simulink model "main"  (R2020b)
settings: Solver=ode23tb  StartTime=0.0  StopTime=20  FixedStep=0.0005  MaxStep=0.005  RelTol=1e-3  AbsTol=1e-3
StartFcn:
  | tic;
StopFcn:
  | Elapsed_Sim_Time = toc;
  | disp(['Elapsed Sim Time = ' num2str(Elapsed_Sim_Time)]);
model workspace (MATLAB code in the model file):
  | floor_l = 1.0900;
  | floor_d = 0.0100;
  | 
  | % PART
  | model_idx = 0;
  | model_dims = [0.06 0.06 0.06;
  |      0.02 0.05 0.07;
  |      0.04 0.04 0.10;
  |      0.05 0.05 0.05;
  |      0.10 0.08 0.08];
  | % distance between models on the conveyor belt
  | model_d = 0.12;
  | % distance to push models forwards in the -y dir (towards the box)
  | model_push = 0.2;
  | 
  | % BELT
  | belt_w = 0.1000;
  | belt_l = 1.2000;
  | belt_h = 0.0200;
  | belt_in_offset = [0 0.8000 0.0100];
  | 
  | container_belt_h = 0.02;
  | container_belt_l = 2.0;
  | container_belt_w = 0.2;
  | container_belt_offset = [-0.5050 0 -0.020];
  | 
  | belt_spd = 0.1;
  | 
  | % Model
  | cube_d = 0.06;
  | cube_z_off = belt_in_offset(3) + (container_belt_h / 2) + 0.001;
  | cube_z_offs = (model_dims(:,3) / 2) + cube_z_off;
  | 
  | % Container dimensions
  | % len, width, height are INTERNAL (Changed because most things were using internal anyway and it's 4am and we just need a working demo)
  | % Dimensions
  | container_len = 0.2;
  | container_width = 0.15;
  | container_height = 0.15;
  | container_thickness = 0.005;
  | 
  | 
  | % ????
  | cube_con_rsph = 0.003;
  | 
  | cube_con_k = 1000000;
  | cube_con_b = 1000;
  | 
  | finger_con_x = 0.01;
  | finger_con_y = 0.01;
  | finger_con_z = 5e-4;
  | finger_con_rsph = 5.0000e-04;
  | finger_con_muk = 0.05;
  | finger_con_mus = 0.07;
  | finger_con_vth = 1e-3;
  | 
  | finger_l = 0.4;
  | finger_w = 0.03;
  | finger_t = 0.01;
undefined symbols (not defined in the file): Bottom, Extr_Data_LinkHoles, Part1, Part2, Part3, Part4, Part5, point1, point2, point3, Side1, Side2, Side3, Side4, X, Y, Z
libraries: sm_lib x113, nesl_utility x35, Parts_Lib x10, Contact_Forces_Lib x6, sm_delta_robot_lib x1
(part 3 of 5)

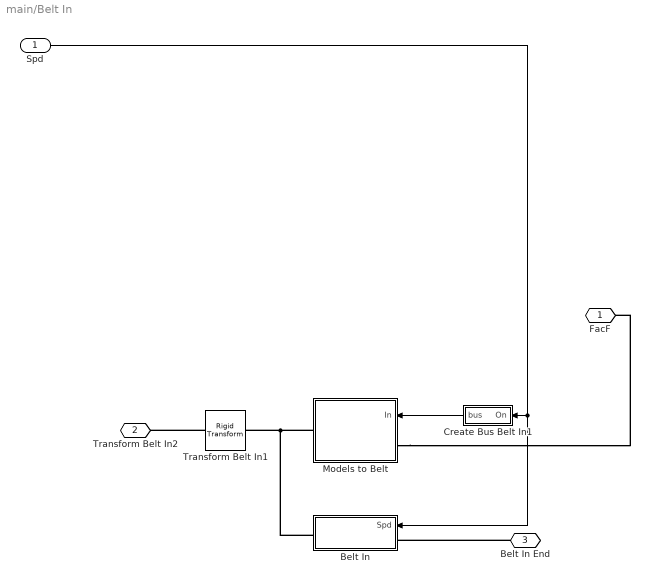
== system main/Belt In ==
  Spd : Inport
  Belt In : Subsystem  Tag=CustomStyle  mask(Conveyor Belt, 5 Rollers){belt_l=belt_l, belt_d=belt_h, belt_w=belt_w, roller_clr=[1 1 1], ctrrefnorm_popup=+Z}
      mask prompts: belt_l "Conveyor Length (m)"; belt_d "Conveyor Depth (m)"; belt_w "Conveyor Width (m)"; roller_clr "Roller Color (rgb)"; ctrrefnorm_popup "Center Reference Frame, Normal Axis"
      mask help: Models a conveyor belt. Input signal is belt speed which only affects roller rotational speed in animation.
      mask init:
      | temp_curblk = gcb;
      | if strcmp(get_param(temp_curblk,'ctrrefnorm_popup'),'+Z')
      |     set_param([temp_curblk '/Transform Contact Ref'],'RotationSequenceAngles','[-90 0 0]');
      | elseif strcmp(get_param(temp_curblk,'ctrrefnorm_popup'),'+X')
      |     set_param([temp_curblk '/Transform Contact Ref'],'RotationSequenceAngles','[0 0 90]');
      | end
      | clear temp_curblk
      mask TypeOptions ctrrefnorm_popup: +Z | +X
  Create Bus Belt In1 : Subsystem
  Models to Belt : Subsystem
  Transform Belt In1 : sm_lib/Frames and Transforms/Rigid Transform  TranslationMethod=Cartesian  TranslationStandardOffset=0  TranslationLengthUnit=m  TranslationStandardAxis=+Y  TranslationCartesianOffset=belt_in_offset  TranslationROffset=0  TranslationROffsetUnits=m  TranslationZOffset=0  TranslationZOffsetUnits=m  TranslationThetaOffset=0  TranslationThetaOffsetUnits=deg  RotationMethod=StandardAxis  RotationAngleUnits=deg  RotationStandardAxis=+Z  RotationAngle=-90  RotationArbitraryAxis=[0 0 1]  FollAlignAxisA=+X  BaseAlignAxisA=+Y  FollAlignAxisB=+Y  BaseAlignAxisB=+Z  RotationSequenceAxes=FollowerAxes  RotationSequence=XYX  RotationSequenceAngles=[0 0 0]  RotationSequenceAnglesUnits=deg  RotationMatrix=[1 0 0; 0 1 0; 0 0 1]
  FacF : PMIOPort  Side=Right
  Transform Belt In2 : PMIOPort  Port=2  Side=Left
  Belt In End : PMIOPort  Port=3  Side=Right
  wires:
  Create Bus Belt In1/1(bus) -> Models to Belt/1(In)
  Spd/1 -> Belt In/1(Spd), Create Bus Belt In1/1(On)
  connections:
  Transform Belt In1/LConn1 -- Transform Belt In2/RConn1
  Models to Belt/RConn1 -- Belt In/RConn1 -- Transform Belt In1/RConn1
  Models to Belt/LConn1 -- FacF/RConn1
  Belt In End/RConn1 -- Belt In/LConn1

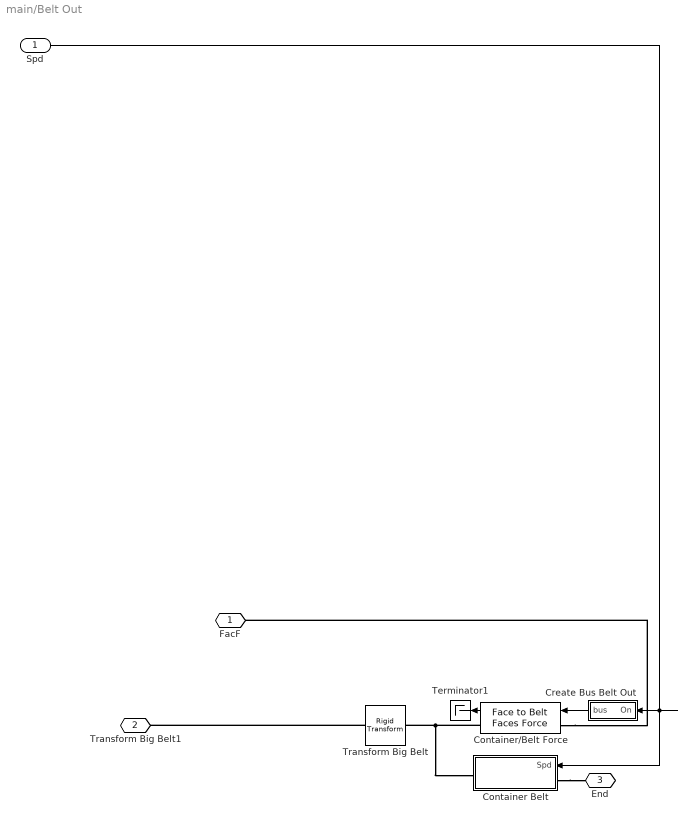
== system main/Belt Out ==
  Spd : Inport
  Container Belt : Subsystem  Tag=CustomStyle  mask(Conveyor Belt, 5 Rollers){belt_l=container_belt_l, belt_d=container_belt_h, belt_w=container_belt_w, roller_clr=[1 1 1], ctrrefnorm_popup=+Z}
      mask prompts: belt_l "Conveyor Length (m)"; belt_d "Conveyor Depth (m)"; belt_w "Conveyor Width (m)"; roller_clr "Roller Color (rgb)"; ctrrefnorm_popup "Center Reference Frame, Normal Axis"
      mask help: Models a conveyor belt. Input signal is belt speed which only affects roller rotational speed in animation.
      mask init: same as main/Belt In/Belt In
      mask TypeOptions ctrrefnorm_popup: +Z | +X
  Container/Belt Force : Contact_Forces_Lib/3D/Composite Forces/Face to Belt Faces Force  PlaB_x=container_belt_l  PlaB_y=container_belt_w  PlaB_z=container_belt_h/2  FacF_x=container_len  FacF_y=container_width  FacF_z=container_thickness/2  FacF_rSph=cube_con_rsph  force_law_pla2pla=Linear  k_contact_pla2pla=stff  b_contact_pla2pla=dmp  pen_full_damp_F_pla2pla=1e-4  pen_exponent_pla2pla=1  friction_law_pla2pla=Stick-Slip Continuous  mu_kinetic_pla2pla=0.5  mu_static_pla2pla=0.7  v_thr_pla2pla=0.001  vis_on_pla2pla=off  vis_opc_en_box2box=0  vis_len_plaLz=0.0005  vis_clr=[0.9 0.2 0.2]  vis_opc=0.7
      link override Sphere to Plane Force Enabled nz1/Forces/Ff/Friction Law/Stick-Slip C /Coefficient of Friction vs Velocity: BeginIndexSearchUsingPreviousIndexResult=on
      link override Sphere to Plane Force Enabled nz2/Forces/Ff/Friction Law/Stick-Slip C /Coefficient of Friction vs Velocity: BeginIndexSearchUsingPreviousIndexResult=on
      link override Sphere to Plane Force Enabled nz3/Forces/Ff/Friction Law/Stick-Slip C /Coefficient of Friction vs Velocity: BeginIndexSearchUsingPreviousIndexResult=on
      settings: SourceProductName=Simscape Multibody Contact Forces Library
  Create Bus Belt Out : Subsystem
  Terminator1 : Terminator
  Transform Big Belt : sm_lib/Frames and Transforms/Rigid Transform  TranslationMethod=Cartesian  TranslationStandardOffset=0  TranslationLengthUnit=m  TranslationStandardAxis=+Y  TranslationCartesianOffset=container_belt_offset  TranslationROffset=0  TranslationROffsetUnits=m  TranslationZOffset=0  TranslationZOffsetUnits=m  TranslationThetaOffset=0  TranslationThetaOffsetUnits=deg  RotationMethod=StandardAxis  RotationAngleUnits=deg  RotationStandardAxis=+Z  RotationAngle=180  RotationArbitraryAxis=[0 0 1]  FollAlignAxisA=+X  BaseAlignAxisA=+Y  FollAlignAxisB=+Y  BaseAlignAxisB=+Z  RotationSequenceAxes=FollowerAxes  RotationSequence=XYX  RotationSequenceAngles=[0 0 0]  RotationSequenceAnglesUnits=deg  RotationMatrix=[1 0 0; 0 1 0; 0 0 1]
  FacF : PMIOPort  Side=Right
  Transform Big Belt1 : PMIOPort  Port=2  Side=Left
  End : PMIOPort  Port=3  Side=Left
  wires:
  Spd/1 -> Container Belt/1(Spd), Create Bus Belt Out/1(On)
  Create Bus Belt Out/1(bus) -> Container/Belt Force/1
  Container/Belt Force/1 -> Terminator1/1
  connections:
  Transform Big Belt/LConn1 -- Transform Big Belt1/RConn1
  Container/Belt Force/RConn1 -- Container Belt/RConn1 -- Transform Big Belt/RConn1
  Container Belt/LConn1 -- End/RConn1
  Container/Belt Force/LConn1 -- FacF/RConn1

== system main/Config ==
  Floor : sm_lib/Body Elements/Brick Solid  Commented=on  GraphicAmbientColor=[0.15 0.15 0.15 1.0]  BasedOnType=Density  BrickDimensions=[floor_l floor_l floor_d]  BrickDimensionUnits=m  CenterOfMass=[0 0 0]  CenterOfMassUnits=m  GraphicDiffuseColor=[0.8 0.8 0.8]  Density=100  DensityUnits=kg/m^3  DoExposeReferenceFrame=on  GraphicEmissiveColor=[0.0 0.0 0.0 1.0]  ExportEntireGeometry=off  SerializedFrames=<Frames><Frame><Id>Frame1</Id><Value><Name>T</Name><Origin><Source>GeometricFeature</Source><FeatureName>+z surface</FeatureName></Origin><PrimaryAxis><DefinedDirection>+Z</DefinedDirection><Source>ReferenceFrame</Source><SourceDirection>+Z</SourceDirection><FeatureName></FeatureName></PrimaryAxis><SecondaryAxis><DefinedDirection>+X</DefinedDirection><Source>ReferenceFrame</Source><SourceDirection>+X</SourceDirection><FeatureName></FeatureName></SecondaryAxis></Value></Frame></Frames>  MarkerShape=Sphere  MarkerSize=10  GraphicType=FromGeometry  InertiaType=CalculateFromGeometry  Mass=1  MassUnits=kg  MomentsOfInertia=[1 1 1]  MomentsOfInertiaUnits=kg*m^2  GraphicOpacity=1.0  ProductsOfInertia=[1 1 1]  ProductsOfInertiaUnits=kg*m^2  GraphicShininess=75  GraphicSpecularColor=[0.5 0.5 0.5 1.0]  GraphicVisPropType=SimpleVisualProperties
  Mechanism Configuration : sm_lib/Utilities/Mechanism Configuration  UniformGravity=Constant  GravityVector=[0 0 -9.80665]  GravityVectorUnits=m/s^2  GravityUnits=m/s^2  LinearizationDelta=0.001  JointModeTransitionNonlinearIterations=2
  Solver Configuration : nesl_utility/Solver Configuration  PhysicalDomain=network_engine_domain  SubClassName=solver  LeftPortType=input  RightPortType=generic  Tones=[]  Harmonics=[]  SimulateNoise=off  Profile=off  UseLocalSampling=off  EnableSwitchedLinearOptims=on  FrequencyDomain=off  UseCCode=off  RelTol=0.001  AbsTol=1e-06  MinStep=1e-09  ToWorkspace=off  RevertToSquareIcSolve=off  NumHomotopyIterations=100  PhasorMode=off  PhasorModeNumHarmonics=1  DoDC=off  ResidualTolerance=1e-05  UseLocalSolver=off  LocalSolverChoice=NE_BACKWARD_EULER_ADVANCER  LocalSolverSampleTime=0.0001  DoFixedCost=off  MaxNonlinIter=3  MaxModeIter=2  ComputeImpulses=on  ImpulseIterations=2  LinearAlgebra=auto  EquationFormulation=NE_TIME_EF  DelaysMemoryBudget=1024  AutomaticFiltering=on  FilteringTimeConstant=0.001  PartitionStorageMethod=AS_NEEDED  PartitionMemoryBudget=1024  PartitionMethod=FAST
  C : PMIOPort  Side=Right
  connections:
  C/RConn1 -- Floor/RConn1 -- Solver Configuration/RConn1 -- Mechanism Configuration/RConn1

== system main/Contacts Models Container ==
  Contacts Model-Container1 : Subsystem  mask{k=500, b=10, mus=0.4, muk=0.4}
      mask prompts: k "Stiffness (N/m)"; b "Dampink (N/(m/s))"; mus "Coefficient of Static Friction"; muk "Coefficient of Dynamic Friction"
      mask DialogControl Control2 Prompt: Force Parameters
  Contacts Model-Container2 : Subsystem  mask{k=500, b=10, mus=0.4, muk=0.4}
      mask prompts: k "Stiffness (N/m)"; b "Dampink (N/(m/s))"; mus "Coefficient of Static Friction"; muk "Coefficient of Dynamic Friction"
      mask DialogControl Control2 Prompt: Force Parameters
  Contacts Model-Container3 : Subsystem  mask{k=500, b=10, mus=0.4, muk=0.4}
      mask prompts: k "Stiffness (N/m)"; b "Dampink (N/(m/s))"; mus "Coefficient of Static Friction"; muk "Coefficient of Dynamic Friction"
      mask DialogControl Control2 Prompt: Force Parameters
  Contacts Model-Container4 : Subsystem  mask{k=500, b=10, mus=0.4, muk=0.4}
      mask prompts: k "Stiffness (N/m)"; b "Dampink (N/(m/s))"; mus "Coefficient of Static Friction"; muk "Coefficient of Dynamic Friction"
      mask DialogControl Control2 Prompt: Force Parameters
  Contacts Model-Container5 : Subsystem  mask{k=500, b=10, mus=0.4, muk=0.4}
      mask prompts: k "Stiffness (N/m)"; b "Dampink (N/(m/s))"; mus "Coefficient of Static Friction"; muk "Coefficient of Dynamic Friction"
      mask DialogControl Control2 Prompt: Force Parameters
  Simscape Bus1 : SimscapeBus  HierarchyStrings=Part1;Part2;Part3;Part4;Part5
  Container : PMIOPort  Side=Left
  Models : PMIOPort  Port=2  Side=Right
  connections:
  Simscape Bus1/RConn1 -- Models/RConn1
  Container/RConn1 -- Contacts Model-Container5/LConn1 -- Contacts Model-Container4/LConn1 -- Contacts Model-Container2/LConn1 -- Contacts Model-Container1/LConn1 -- Contacts Model-Container3/LConn1
  Contacts Model-Container1/RConn1 -- Simscape Bus1/LConn1
  Contacts Model-Container2/RConn1 -- Simscape Bus1/LConn2
  Contacts Model-Container3/RConn1 -- Simscape Bus1/LConn3
  Contacts Model-Container4/RConn1 -- Simscape Bus1/LConn4
  Contacts Model-Container5/RConn1 -- Simscape Bus1/LConn5

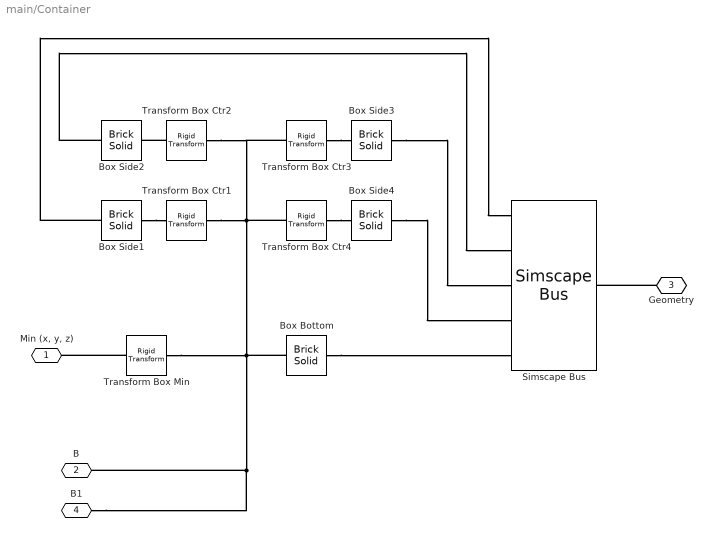
== system main/Container ==
  Box Bottom : sm_lib/Body Elements/Brick Solid  GraphicAmbientColor=[0.15 0.15 0.15 1.0]  BasedOnType=Density  BrickDimensions=[box_l+2*box_wt box_w+2*box_wt box_wt]  BrickDimensionUnits=m  CenterOfMass=[0 0 0]  CenterOfMassUnits=m  GraphicDiffuseColor=box_color  Density=1000  DensityUnits=kg/(m^3)  DoExposeReferenceFrame=on  GraphicEmissiveColor=[0.0 0.0 0.0 1.0]  ExportEntireGeometry=on  SerializedFrames=<Frames/>  MarkerShape=Sphere  MarkerSize=10  GraphicType=FromGeometry  InertiaType=CalculateFromGeometry  Mass=1  MassUnits=kg  MomentsOfInertia=[1 1 1]  MomentsOfInertiaUnits=kg*m^2  GraphicOpacity=box_opacity  ProductsOfInertia=[0 0 0]  ProductsOfInertiaUnits=kg*m^2  GraphicShininess=75  GraphicSpecularColor=[0.5 0.5 0.5 1.0]  GraphicVisPropType=SimpleVisualProperties
  Box Side1 : sm_lib/Body Elements/Brick Solid  GraphicAmbientColor=[0.15 0.15 0.15 1.0]  BasedOnType=Density  BrickDimensions=[box_l+2*box_wt box_wt box_h + 2*box_wt]  BrickDimensionUnits=m  CenterOfMass=[0 0 0]  CenterOfMassUnits=m  GraphicDiffuseColor=box_color  Density=1000  DensityUnits=kg/(m^3)  DoExposeReferenceFrame=on  GraphicEmissiveColor=[0.0 0.0 0.0 1.0]  ExportEntireGeometry=on  SerializedFrames=<Frames/>  MarkerShape=Sphere  MarkerSize=10  GraphicType=FromGeometry  InertiaType=CalculateFromGeometry  Mass=1  MassUnits=kg  MomentsOfInertia=[1 1 1]  MomentsOfInertiaUnits=kg*m^2  GraphicOpacity=box_opacity  ProductsOfInertia=[0 0 0]  ProductsOfInertiaUnits=kg*m^2  GraphicShininess=75  GraphicSpecularColor=[0.5 0.5 0.5 1.0]  GraphicVisPropType=SimpleVisualProperties
  Box Side2 : sm_lib/Body Elements/Brick Solid  GraphicAmbientColor=[0.15 0.15 0.15 1.0]  BasedOnType=Density  BrickDimensions=[box_l+2*box_wt box_wt box_h+ 2*box_wt]  BrickDimensionUnits=m  CenterOfMass=[0 0 0]  CenterOfMassUnits=m  GraphicDiffuseColor=box_color  Density=1000  DensityUnits=kg/(m^3)  DoExposeReferenceFrame=on  GraphicEmissiveColor=[0.0 0.0 0.0 1.0]  ExportEntireGeometry=on  SerializedFrames=<Frames/>  MarkerShape=Sphere  MarkerSize=10  GraphicType=FromGeometry  InertiaType=CalculateFromGeometry  Mass=1  MassUnits=kg  MomentsOfInertia=[1 1 1]  MomentsOfInertiaUnits=kg*m^2  GraphicOpacity=box_opacity  ProductsOfInertia=[0 0 0]  ProductsOfInertiaUnits=kg*m^2  GraphicShininess=75  GraphicSpecularColor=[0.5 0.5 0.5 1.0]  GraphicVisPropType=SimpleVisualProperties
  Box Side3 : sm_lib/Body Elements/Brick Solid  GraphicAmbientColor=[0.15 0.15 0.15 1.0]  BasedOnType=Density  BrickDimensions=[box_wt box_w+2*box_wt box_h + 2*box_wt]  BrickDimensionUnits=m  CenterOfMass=[0 0 0]  CenterOfMassUnits=m  GraphicDiffuseColor=box_color  Density=1000  DensityUnits=kg/(m^3)  DoExposeReferenceFrame=on  GraphicEmissiveColor=[0.0 0.0 0.0 1.0]  ExportEntireGeometry=on  SerializedFrames=<Frames/>  MarkerShape=Sphere  MarkerSize=10  GraphicType=FromGeometry  InertiaType=CalculateFromGeometry  Mass=1  MassUnits=kg  MomentsOfInertia=[1 1 1]  MomentsOfInertiaUnits=kg*m^2  GraphicOpacity=box_opacity  ProductsOfInertia=[0 0 0]  ProductsOfInertiaUnits=kg*m^2  GraphicShininess=75  GraphicSpecularColor=[0.5 0.5 0.5 1.0]  GraphicVisPropType=SimpleVisualProperties
  Box Side4 : sm_lib/Body Elements/Brick Solid  GraphicAmbientColor=[0.15 0.15 0.15 1.0]  BasedOnType=Density  BrickDimensions=[box_wt box_w+2*box_wt box_h + 2*box_wt]  BrickDimensionUnits=m  CenterOfMass=[0 0 0]  CenterOfMassUnits=m  GraphicDiffuseColor=box_color  Density=1000  DensityUnits=kg/(m^3)  DoExposeReferenceFrame=on  GraphicEmissiveColor=[0.0 0.0 0.0 1.0]  ExportEntireGeometry=on  SerializedFrames=<Frames/>  MarkerShape=Sphere  MarkerSize=10  GraphicType=FromGeometry  InertiaType=CalculateFromGeometry  Mass=1  MassUnits=kg  MomentsOfInertia=[1 1 1]  MomentsOfInertiaUnits=kg*m^2  GraphicOpacity=box_opacity  ProductsOfInertia=[0 0 0]  ProductsOfInertiaUnits=kg*m^2  GraphicShininess=75  GraphicSpecularColor=[0.5 0.5 0.5 1.0]  GraphicVisPropType=SimpleVisualProperties
  Simscape Bus : SimscapeBus  HierarchyStrings=Side1;Side2;Side3;Side4;Bottom
  Transform Box Ctr1 : sm_lib/Frames and Transforms/Rigid Transform  TranslationMethod=Cartesian  TranslationStandardOffset=box_h/2+box_wt/2  TranslationLengthUnit=m  TranslationStandardAxis=+Z  TranslationCartesianOffset=[0 (box_w + box_wt)/2 -(box_h + box_wt)/2]  TranslationROffset=0  TranslationROffsetUnits=m  TranslationZOffset=0  TranslationZOffsetUnits=m  TranslationThetaOffset=0  TranslationThetaOffsetUnits=deg  RotationMethod=None  RotationAngleUnits=deg  RotationStandardAxis=+Z  RotationAngle=0.0  RotationArbitraryAxis=[0 0 1]  FollAlignAxisA=+X  BaseAlignAxisA=+Y  FollAlignAxisB=+Y  BaseAlignAxisB=+Z  RotationSequenceAxes=FollowerAxes  RotationSequence=XYX  RotationSequenceAngles=[0 0 0]  RotationSequenceAnglesUnits=deg  RotationMatrix=[1 0 0; 0 1 0; 0 0 1]
  Transform Box Ctr2 : sm_lib/Frames and Transforms/Rigid Transform  TranslationMethod=Cartesian  TranslationStandardOffset=box_h/2+box_wt/2  TranslationLengthUnit=m  TranslationStandardAxis=+Z  TranslationCartesianOffset=[0 -(box_w+box_wt)/2 -(box_h + box_wt)/2]  TranslationROffset=0  TranslationROffsetUnits=m  TranslationZOffset=0  TranslationZOffsetUnits=m  TranslationThetaOffset=0  TranslationThetaOffsetUnits=deg  RotationMethod=None  RotationAngleUnits=deg  RotationStandardAxis=+Z  RotationAngle=0.0  RotationArbitraryAxis=[0 0 1]  FollAlignAxisA=+X  BaseAlignAxisA=+Y  FollAlignAxisB=+Y  BaseAlignAxisB=+Z  RotationSequenceAxes=FollowerAxes  RotationSequence=XYX  RotationSequenceAngles=[0 0 0]  RotationSequenceAnglesUnits=deg  RotationMatrix=[1 0 0; 0 1 0; 0 0 1]
  Transform Box Ctr3 : sm_lib/Frames and Transforms/Rigid Transform  TranslationMethod=Cartesian  TranslationStandardOffset=box_h/2+box_wt/2  TranslationLengthUnit=m  TranslationStandardAxis=+Z  TranslationCartesianOffset=[(box_l+box_wt)/2 0 (box_h+box_wt)/2]  TranslationROffset=0  TranslationROffsetUnits=m  TranslationZOffset=0  TranslationZOffsetUnits=m  TranslationThetaOffset=0  TranslationThetaOffsetUnits=deg  RotationMethod=None  RotationAngleUnits=deg  RotationStandardAxis=+Z  RotationAngle=0.0  RotationArbitraryAxis=[0 0 1]  FollAlignAxisA=+X  BaseAlignAxisA=+Y  FollAlignAxisB=+Y  BaseAlignAxisB=+Z  RotationSequenceAxes=FollowerAxes  RotationSequence=XYX  RotationSequenceAngles=[0 0 0]  RotationSequenceAnglesUnits=deg  RotationMatrix=[1 0 0; 0 1 0; 0 0 1]
  Transform Box Ctr4 : sm_lib/Frames and Transforms/Rigid Transform  TranslationMethod=Cartesian  TranslationStandardOffset=box_h/2+box_wt/2  TranslationLengthUnit=m  TranslationStandardAxis=+Z  TranslationCartesianOffset=[-(box_l/2+box_wt/2) 0 box_h/2+box_wt/2]  TranslationROffset=0  TranslationROffsetUnits=m  TranslationZOffset=0  TranslationZOffsetUnits=m  TranslationThetaOffset=0  TranslationThetaOffsetUnits=deg  RotationMethod=None  RotationAngleUnits=deg  RotationStandardAxis=+Z  RotationAngle=0.0  RotationArbitraryAxis=[0 0 1]  FollAlignAxisA=+X  BaseAlignAxisA=+Y  FollAlignAxisB=+Y  BaseAlignAxisB=+Z  RotationSequenceAxes=FollowerAxes  RotationSequence=XYX  RotationSequenceAngles=[0 0 0]  RotationSequenceAnglesUnits=deg  RotationMatrix=[1 0 0; 0 1 0; 0 0 1]
  Transform Box Min : sm_lib/Frames and Transforms/Rigid Transform  TranslationMethod=Cartesian  TranslationStandardOffset=box_h/2+box_wt/2  TranslationLengthUnit=m  TranslationStandardAxis=+Z  TranslationCartesianOffset=[box_l/2 + box_wt, box_w/2 + box_wt, -box_wt/2]  TranslationROffset=0  TranslationROffsetUnits=m  TranslationZOffset=0  TranslationZOffsetUnits=m  TranslationThetaOffset=0  TranslationThetaOffsetUnits=deg  RotationMethod=None  RotationAngleUnits=deg  RotationStandardAxis=+Z  RotationAngle=0.0  RotationArbitraryAxis=[0 0 1]  FollAlignAxisA=+X  BaseAlignAxisA=+Y  FollAlignAxisB=+Y  BaseAlignAxisB=+Z  RotationSequenceAxes=FollowerAxes  RotationSequence=XYX  RotationSequenceAngles=[0 0 0]  RotationSequenceAnglesUnits=deg  RotationMatrix=[1 0 0; 0 1 0; 0 0 1]
  "Min (x, y, z)" : PMIOPort  Side=Left
  B : PMIOPort  Port=2  Side=Left
  Geometry : PMIOPort  Port=3  Side=Right
  B1 : PMIOPort  Port=4  Side=Right
  connections:
  Box Bottom/RConn1 -- Transform Box Min/LConn1 -- Transform Box Ctr1/RConn1 -- Transform Box Ctr2/RConn1 -- Transform Box Ctr3/LConn1 -- Transform Box Ctr4/LConn1 -- B1/RConn1 -- B/RConn1
  Transform Box Ctr3/RConn1 -- Box Side3/RConn1
  Transform Box Ctr4/RConn1 -- Box Side4/RConn1
  Transform Box Ctr2/LConn1 -- Box Side2/RConn1
  Box Side1/RConn1 -- Transform Box Ctr1/LConn1
  Geometry/RConn1 -- Simscape Bus/RConn1
  Box Bottom/LConn1 -- Simscape Bus/LConn5
  Box Side1/LConn1 -- Simscape Bus/LConn1
  Box Side2/LConn1 -- Simscape Bus/LConn2
  Box Side3/LConn1 -- Simscape Bus/LConn3
  Box Side4/LConn1 -- Simscape Bus/LConn4
  Transform Box Min/RConn1 -- "Min (x, y, z)"/RConn1

== system main/End Effector-Part Contact Forces1 ==
  End Effector Part 1 : Subsystem  mask(End Effector-Part Contact Forces){k=1e6, b=10, mus=0.4, muk=0.4}
      mask prompts: k "Stiffness (N/m)"; b "Damping (N/(m/s))"; mus "Coefficient of Static Friction"; muk "Coefficient of Dynamic Friction"
      mask help: This block models the contact forces between the end effector and the part. The entire cylindrical part geometry is used, but the end effector geometry corresponds to the three contact points around the tip.
  End Effector Part 2 : Subsystem  mask(End Effector-Part Contact Forces){k=1e6, b=10, mus=0.4, muk=0.4}
      mask prompts: k "Stiffness (N/m)"; b "Damping (N/(m/s))"; mus "Coefficient of Static Friction"; muk "Coefficient of Dynamic Friction"
      mask help: This block models the contact forces between the end effector and the part. The entire cylindrical part geometry is used, but the end effector geometry corresponds to the three contact points around the tip.
  End Effector Part 3 : Subsystem  mask(End Effector-Part Contact Forces){k=1e6, b=10, mus=0.4, muk=0.4}
      mask prompts: k "Stiffness (N/m)"; b "Damping (N/(m/s))"; mus "Coefficient of Static Friction"; muk "Coefficient of Dynamic Friction"
      mask help: This block models the contact forces between the end effector and the part. The entire cylindrical part geometry is used, but the end effector geometry corresponds to the three contact points around the tip.
  End Effector Part 4 : Subsystem  mask(End Effector-Part Contact Forces){k=1e6, b=10, mus=0.4, muk=0.4}
      mask prompts: k "Stiffness (N/m)"; b "Damping (N/(m/s))"; mus "Coefficient of Static Friction"; muk "Coefficient of Dynamic Friction"
      mask help: This block models the contact forces between the end effector and the part. The entire cylindrical part geometry is used, but the end effector geometry corresponds to the three contact points around the tip.
  End Effector Part 5 : Subsystem  mask(End Effector-Part Contact Forces){k=1e6, b=10, mus=0.4, muk=0.4}
      mask prompts: k "Stiffness (N/m)"; b "Damping (N/(m/s))"; mus "Coefficient of Static Friction"; muk "Coefficient of Dynamic Friction"
      mask help: This block models the contact forces between the end effector and the part. The entire cylindrical part geometry is used, but the end effector geometry corresponds to the three contact points around the tip.
  Simscape Bus2 : SimscapeBus  HierarchyStrings=Part1;Part2;Part3;Part4;Part5
  End Effector : PMIOPort  Side=Left
  Models : PMIOPort  Port=2  Side=Right
  connections:
  End Effector/RConn1 -- End Effector Part 3/LConn1 -- End Effector Part 2/LConn1 -- End Effector Part 1/LConn1 -- End Effector Part 5/LConn1 -- End Effector Part 4/LConn1
  End Effector Part 1/RConn1 -- Simscape Bus2/LConn1
  End Effector Part 2/RConn1 -- Simscape Bus2/LConn2
  End Effector Part 3/RConn1 -- Simscape Bus2/LConn3
  End Effector Part 4/RConn1 -- Simscape Bus2/LConn4
  Simscape Bus2/LConn5 -- End Effector Part 5/RConn1
  Simscape Bus2/RConn1 -- Models/RConn1

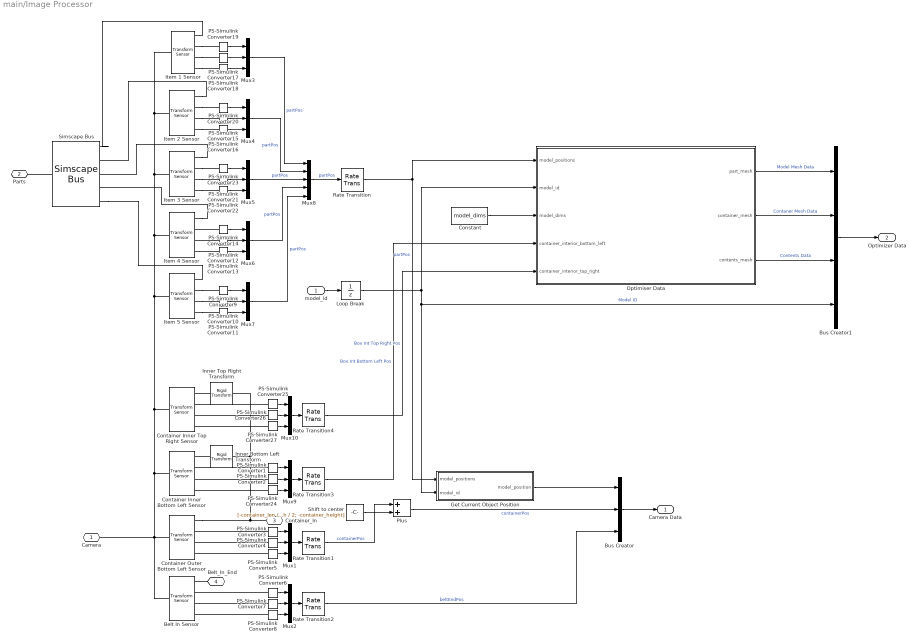
== system main/Image Processor ==
  model_id : Inport
  Belt In Sensor : sm_lib/Frames and Transforms/Transform Sensor  MeasurementFrame=Base  SenseAngle=off  SenseAxis=off  SenseAngle1=off  SenseAngle2=off  SenseAngle3=off  SenseQ=off  SenseR=off  SenseOmegaX=off  SenseOmegaY=off  SenseOmegaZ=off  SenseOmega1=off  SenseOmega2=off  SenseOmega3=off  SenseQDot=off  SenseRDot=off  SenseAlphaX=off  SenseAlphaY=off  SenseAlphaZ=off  SenseAlpha1=off  SenseAlpha2=off  SenseAlpha3=off  SenseQDDot=off  SenseRDDot=off  SenseX=on  SenseY=on  SenseZ=on  SenseRad=off  SenseAzim=off  SenseDist=off  SenseInc=off  SenseXDot=off  SenseYDot=off  SenseZDot=off  SenseRadDot=off  SenseAzimDot=off  SenseDistDot=off  SenseIncDot=off  SenseXDDot=off  SenseYDDot=off  SenseZDDot=off  SenseRadDDot=off  SenseAzimDDot=off  SenseDistDDot=off  SenseIncDDot=off
  Bus Creator : BusCreator  Inputs=3  OutDataTypeStr=Bus: cam_data
  Bus Creator1 : BusCreator  Inputs=4
  Constant : Constant  Value=model_dims  VectorParams1D=off
  Container Inner Bottom Left Sensor : sm_lib/Frames and Transforms/Transform Sensor  MeasurementFrame=Base  SenseAngle=off  SenseAxis=off  SenseAngle1=off  SenseAngle2=off  SenseAngle3=off  SenseQ=off  SenseR=off  SenseOmegaX=off  SenseOmegaY=off  SenseOmegaZ=off  SenseOmega1=off  SenseOmega2=off  SenseOmega3=off  SenseQDot=off  SenseRDot=off  SenseAlphaX=off  SenseAlphaY=off  SenseAlphaZ=off  SenseAlpha1=off  SenseAlpha2=off  SenseAlpha3=off  SenseQDDot=off  SenseRDDot=off  SenseX=on  SenseY=on  SenseZ=on  SenseRad=off  SenseAzim=off  SenseDist=off  SenseInc=off  SenseXDot=off  SenseYDot=off  SenseZDot=off  SenseRadDot=off  SenseAzimDot=off  SenseDistDot=off  SenseIncDot=off  SenseXDDot=off  SenseYDDot=off  SenseZDDot=off  SenseRadDDot=off  SenseAzimDDot=off  SenseDistDDot=off  SenseIncDDot=off
      settings: SourceProductName=Multibody
  Container Inner Top Right Sensor : sm_lib/Frames and Transforms/Transform Sensor  MeasurementFrame=Base  SenseAngle=off  SenseAxis=off  SenseAngle1=off  SenseAngle2=off  SenseAngle3=off  SenseQ=off  SenseR=off  SenseOmegaX=off  SenseOmegaY=off  SenseOmegaZ=off  SenseOmega1=off  SenseOmega2=off  SenseOmega3=off  SenseQDot=off  SenseRDot=off  SenseAlphaX=off  SenseAlphaY=off  SenseAlphaZ=off  SenseAlpha1=off  SenseAlpha2=off  SenseAlpha3=off  SenseQDDot=off  SenseRDDot=off  SenseX=on  SenseY=on  SenseZ=on  SenseRad=off  SenseAzim=off  SenseDist=off  SenseInc=off  SenseXDot=off  SenseYDot=off  SenseZDot=off  SenseRadDot=off  SenseAzimDot=off  SenseDistDot=off  SenseIncDot=off  SenseXDDot=off  SenseYDDot=off  SenseZDDot=off  SenseRadDDot=off  SenseAzimDDot=off  SenseDistDDot=off  SenseIncDDot=off
      settings: SourceProductName=Multibody
  Container Outer Bottom Left Sensor : sm_lib/Frames and Transforms/Transform Sensor  MeasurementFrame=Base  SenseAngle=off  SenseAxis=off  SenseAngle1=off  SenseAngle2=off  SenseAngle3=off  SenseQ=off  SenseR=off  SenseOmegaX=off  SenseOmegaY=off  SenseOmegaZ=off  SenseOmega1=off  SenseOmega2=off  SenseOmega3=off  SenseQDot=off  SenseRDot=off  SenseAlphaX=off  SenseAlphaY=off  SenseAlphaZ=off  SenseAlpha1=off  SenseAlpha2=off  SenseAlpha3=off  SenseQDDot=off  SenseRDDot=off  SenseX=on  SenseY=on  SenseZ=on  SenseRad=off  SenseAzim=off  SenseDist=off  SenseInc=off  SenseXDot=off  SenseYDot=off  SenseZDot=off  SenseRadDot=off  SenseAzimDot=off  SenseDistDot=off  SenseIncDot=off  SenseXDDot=off  SenseYDDot=off  SenseZDDot=off  SenseRadDDot=off  SenseAzimDDot=off  SenseDistDDot=off  SenseIncDDot=off
      settings: SourceProductName=Multibody
  Get Current Object Position : MATLAB Function  TreatAsAtomicUnit=on
  Inner Bottom Left Transform : sm_lib/Frames and Transforms/Rigid Transform  TranslationMethod=Cartesian  TranslationStandardOffset=0  TranslationLengthUnit=m  TranslationStandardAxis=+Z  TranslationCartesianOffset=[-container_thickness, -container_thickness, container_thickness]  TranslationROffset=0  TranslationROffsetUnits=m  TranslationZOffset=0  TranslationZOffsetUnits=m  TranslationThetaOffset=0  TranslationThetaOffsetUnits=deg  RotationMethod=None  RotationAngleUnits=deg  RotationStandardAxis=+Z  RotationAngle=0.0  RotationArbitraryAxis=[0 0 1]  FollAlignAxisA=+X  BaseAlignAxisA=+Y  FollAlignAxisB=+Y  BaseAlignAxisB=+Z  RotationSequenceAxes=FollowerAxes  RotationSequence=XYX  RotationSequenceAngles=[0 0 0]  RotationSequenceAnglesUnits=deg  RotationMatrix=[1 0 0; 0 1 0; 0 0 1]
  Inner Top Right Transform : sm_lib/Frames and Transforms/Rigid Transform  TranslationMethod=Cartesian  TranslationStandardOffset=0  TranslationLengthUnit=m  TranslationStandardAxis=+Z  TranslationCartesianOffset=[-(container_len + container_thickness), -(container_width + container_thickness), container_height + 2*container_thickness]  TranslationROffset=0  TranslationROffsetUnits=m  TranslationZOffset=0  TranslationZOffsetUnits=m  TranslationThetaOffset=0  TranslationThetaOffsetUnits=deg  RotationMethod=None  RotationAngleUnits=deg  RotationStandardAxis=+Z  RotationAngle=0.0  RotationArbitraryAxis=[0 0 1]  FollAlignAxisA=+X  BaseAlignAxisA=+Y  FollAlignAxisB=+Y  BaseAlignAxisB=+Z  RotationSequenceAxes=FollowerAxes  RotationSequence=XYX  RotationSequenceAngles=[0 0 0]  RotationSequenceAnglesUnits=deg  RotationMatrix=[1 0 0; 0 1 0; 0 0 1]
  Item 1 Sensor : sm_lib/Frames and Transforms/Transform Sensor  MeasurementFrame=World  SenseAngle=off  SenseAxis=off  SenseAngle1=off  SenseAngle2=off  SenseAngle3=off  SenseQ=off  SenseR=off  SenseOmegaX=off  SenseOmegaY=off  SenseOmegaZ=off  SenseOmega1=off  SenseOmega2=off  SenseOmega3=off  SenseQDot=off  SenseRDot=off  SenseAlphaX=off  SenseAlphaY=off  SenseAlphaZ=off  SenseAlpha1=off  SenseAlpha2=off  SenseAlpha3=off  SenseQDDot=off  SenseRDDot=off  SenseX=on  SenseY=on  SenseZ=on  SenseRad=off  SenseAzim=off  SenseDist=off  SenseInc=off  SenseXDot=off  SenseYDot=off  SenseZDot=off  SenseRadDot=off  SenseAzimDot=off  SenseDistDot=off  SenseIncDot=off  SenseXDDot=off  SenseYDDot=off  SenseZDDot=off  SenseRadDDot=off  SenseAzimDDot=off  SenseDistDDot=off  SenseIncDDot=off
      settings: SourceProductName=Multibody
  Item 2 Sensor : sm_lib/Frames and Transforms/Transform Sensor  MeasurementFrame=World  SenseAngle=off  SenseAxis=off  SenseAngle1=off  SenseAngle2=off  SenseAngle3=off  SenseQ=off  SenseR=off  SenseOmegaX=off  SenseOmegaY=off  SenseOmegaZ=off  SenseOmega1=off  SenseOmega2=off  SenseOmega3=off  SenseQDot=off  SenseRDot=off  SenseAlphaX=off  SenseAlphaY=off  SenseAlphaZ=off  SenseAlpha1=off  SenseAlpha2=off  SenseAlpha3=off  SenseQDDot=off  SenseRDDot=off  SenseX=on  SenseY=on  SenseZ=on  SenseRad=off  SenseAzim=off  SenseDist=off  SenseInc=off  SenseXDot=off  SenseYDot=off  SenseZDot=off  SenseRadDot=off  SenseAzimDot=off  SenseDistDot=off  SenseIncDot=off  SenseXDDot=off  SenseYDDot=off  SenseZDDot=off  SenseRadDDot=off  SenseAzimDDot=off  SenseDistDDot=off  SenseIncDDot=off
      settings: SourceProductName=Multibody
  Item 3 Sensor : sm_lib/Frames and Transforms/Transform Sensor  MeasurementFrame=World  SenseAngle=off  SenseAxis=off  SenseAngle1=off  SenseAngle2=off  SenseAngle3=off  SenseQ=off  SenseR=off  SenseOmegaX=off  SenseOmegaY=off  SenseOmegaZ=off  SenseOmega1=off  SenseOmega2=off  SenseOmega3=off  SenseQDot=off  SenseRDot=off  SenseAlphaX=off  SenseAlphaY=off  SenseAlphaZ=off  SenseAlpha1=off  SenseAlpha2=off  SenseAlpha3=off  SenseQDDot=off  SenseRDDot=off  SenseX=on  SenseY=on  SenseZ=on  SenseRad=off  SenseAzim=off  SenseDist=off  SenseInc=off  SenseXDot=off  SenseYDot=off  SenseZDot=off  SenseRadDot=off  SenseAzimDot=off  SenseDistDot=off  SenseIncDot=off  SenseXDDot=off  SenseYDDot=off  SenseZDDot=off  SenseRadDDot=off  SenseAzimDDot=off  SenseDistDDot=off  SenseIncDDot=off
      settings: SourceProductName=Multibody
  Item 4 Sensor : sm_lib/Frames and Transforms/Transform Sensor  MeasurementFrame=World  SenseAngle=off  SenseAxis=off  SenseAngle1=off  SenseAngle2=off  SenseAngle3=off  SenseQ=off  SenseR=off  SenseOmegaX=off  SenseOmegaY=off  SenseOmegaZ=off  SenseOmega1=off  SenseOmega2=off  SenseOmega3=off  SenseQDot=off  SenseRDot=off  SenseAlphaX=off  SenseAlphaY=off  SenseAlphaZ=off  SenseAlpha1=off  SenseAlpha2=off  SenseAlpha3=off  SenseQDDot=off  SenseRDDot=off  SenseX=on  SenseY=on  SenseZ=on  SenseRad=off  SenseAzim=off  SenseDist=off  SenseInc=off  SenseXDot=off  SenseYDot=off  SenseZDot=off  SenseRadDot=off  SenseAzimDot=off  SenseDistDot=off  SenseIncDot=off  SenseXDDot=off  SenseYDDot=off  SenseZDDot=off  SenseRadDDot=off  SenseAzimDDot=off  SenseDistDDot=off  SenseIncDDot=off
      settings: SourceProductName=Multibody
  Item 5 Sensor : sm_lib/Frames and Transforms/Transform Sensor  MeasurementFrame=World  SenseAngle=off  SenseAxis=off  SenseAngle1=off  SenseAngle2=off  SenseAngle3=off  SenseQ=off  SenseR=off  SenseOmegaX=off  SenseOmegaY=off  SenseOmegaZ=off  SenseOmega1=off  SenseOmega2=off  SenseOmega3=off  SenseQDot=off  SenseRDot=off  SenseAlphaX=off  SenseAlphaY=off  SenseAlphaZ=off  SenseAlpha1=off  SenseAlpha2=off  SenseAlpha3=off  SenseQDDot=off  SenseRDDot=off  SenseX=on  SenseY=on  SenseZ=on  SenseRad=off  SenseAzim=off  SenseDist=off  SenseInc=off  SenseXDot=off  SenseYDot=off  SenseZDot=off  SenseRadDot=off  SenseAzimDot=off  SenseDistDot=off  SenseIncDot=off  SenseXDDot=off  SenseYDDot=off  SenseZDDot=off  SenseRadDDot=off  SenseAzimDDot=off  SenseDistDDot=off  SenseIncDDot=off
      settings: SourceProductName=Multibody
  Loop Break : UnitDelay  InitialCondition=1  SampleTime=-1  HasFrameUpgradeWarning=on
  Mux{1..7,9..10} (9 alike) : Mux  Inputs=3
  Mux8 : Mux  Inputs=5
  Optimiser Data : MATLAB Function  TreatAsAtomicUnit=on
  PS-Simulink Converter{1..27} (27 alike) : nesl_utility/PS-Simulink Converter  PhysicalDomain=network_engine_domain  SubClassName=ps_output  LeftPortType=input  RightPortType=output  PseudoPeriodic=off  Frequencies=[]  Unit=m  AffineConversion=off
      settings: SourceProductName=Utilities
  Plus : Sum
  Rate Transition{,1..4} (5 alike) : RateTransition
  Shift to center : Constant  Value=[-container_len / 2; container_width / 2; -container_height]  VectorParams1D=off
  Simscape Bus : SimscapeBus  HierarchyStrings=Part1;Part2;Part3;Part4;Part5
  Camera : PMIOPort  Side=Left
  Parts : PMIOPort  Port=2  Side=Left
  Container_In : PMIOPort  Port=3  Side=Left
  Belt_In_End : PMIOPort  Port=4  Side=Left
  Camera Data : Outport
  Optimizer Data : Outport  Port=2
  wires:
  PS-Simulink Converter3/1 -> Mux1/1
  PS-Simulink Converter5/1 -> Mux1/3
  PS-Simulink Converter4/1 -> Mux1/2
  Mux1/1 -> Rate Transition1/1
  PS-Simulink Converter7/1 -> Mux2/2
  PS-Simulink Converter8/1 -> Mux2/3
  PS-Simulink Converter6/1 -> Mux2/1
  PS-Simulink Converter9/1 -> Mux7/1
  PS-Simulink Converter10/1 -> Mux7/2
  PS-Simulink Converter11/1 -> Mux7/3
  PS-Simulink Converter14/1 -> Mux6/1
  PS-Simulink Converter13/1 -> Mux6/3
  PS-Simulink Converter12/1 -> Mux6/2
  PS-Simulink Converter15/1 -> Mux4/2
  PS-Simulink Converter18/1 -> Mux3/3
  PS-Simulink Converter17/1 -> Mux3/2
  PS-Simulink Converter19/1 -> Mux3/1
  PS-Simulink Converter20/1 -> Mux4/1
  PS-Simulink Converter16/1 -> Mux4/3
  PS-Simulink Converter23/1 -> Mux5/1
  PS-Simulink Converter22/1 -> Mux5/3
  PS-Simulink Converter21/1 -> Mux5/2
  Mux3/1 -> Mux8/1  "partPos"
  Mux4/1 -> Mux8/2  "partPos"
  Mux5/1 -> Mux8/3  "partPos"
  Mux6/1 -> Mux8/4  "partPos"
  Mux7/1 -> Mux8/5  "partPos"
  Mux8/1 -> Rate Transition/1  "partPos"
  Get Current Object Position/1(model_position) -> Bus Creator/1
  Mux2/1 -> Rate Transition2/1
  Optimiser Data/1(part_mesh) -> Bus Creator1/1  "Model Mesh Data"
  Optimiser Data/2(container_mesh) -> Bus Creator1/2  "Contaner Mesh Data"
  Optimiser Data/3(contents_mesh) -> Bus Creator1/3  "Contents Data"
  Bus Creator1/1 -> Optimizer Data/1
  Bus Creator/1 -> Camera Data/1
  model_id/1 -> Loop Break/1
  Plus/1 -> Bus Creator/2  "containerPos"
  Shift to center/1 -> Plus/2
  Rate Transition2/1 -> Bus Creator/3  "beltEndPos"
  Loop Break/1 -> Optimiser Data/2(model_id), Get Current Object Position/2(model_id), Bus Creator1/4  "Model ID"
  Constant/1 -> Optimiser Data/3(model_dims)
  Rate Transition/1 -> Optimiser Data/1(model_positions), Get Current Object Position/1(model_positions)  "partPos"
  Rate Transition1/1 -> Plus/1  "containerPos"
  PS-Simulink Converter2/1 -> Mux9/2
  PS-Simulink Converter24/1 -> Mux9/3
  Mux9/1 -> Rate Transition3/1
  PS-Simulink Converter1/1 -> Mux9/1
  Rate Transition3/1 -> Optimiser Data/4(container_interior_bottom_left)  "Box Int Bottom Left Pos"
  Mux10/1 -> Rate Transition4/1
  PS-Simulink Converter27/1 -> Mux10/3
  PS-Simulink Converter26/1 -> Mux10/2
  PS-Simulink Converter25/1 -> Mux10/1
  Rate Transition4/1 -> Optimiser Data/5(container_interior_top_right)  "Box Int Top Right Pos"
  connections:
  PS-Simulink Converter4/LConn1 -- Container Outer Bottom Left Sensor/RConn3
  PS-Simulink Converter5/LConn1 -- Container Outer Bottom Left Sensor/RConn4
  PS-Simulink Converter3/LConn1 -- Container Outer Bottom Left Sensor/RConn2
  Container Outer Bottom Left Sensor/RConn1 -- Container_In/RConn1 -- Inner Top Right Transform/LConn1 -- Inner Bottom Left Transform/LConn1
  Camera/RConn1 -- Item 1 Sensor/LConn1 -- Item 2 Sensor/LConn1 -- Item 3 Sensor/LConn1 -- Item 4 Sensor/LConn1 -- Item 5 Sensor/LConn1 -- Container Inner Top Right Sensor/LConn1 -- Container Inner Bottom Left Sensor/LConn1 -- Container Outer Bottom Left Sensor/LConn1 -- Belt In Sensor/LConn1
  PS-Simulink Converter7/LConn1 -- Belt In Sensor/RConn3
  Belt_In_End/RConn1 -- Belt In Sensor/RConn1
  PS-Simulink Converter6/LConn1 -- Belt In Sensor/RConn2
  PS-Simulink Converter8/LConn1 -- Belt In Sensor/RConn4
  Item 5 Sensor/RConn2 -- PS-Simulink Converter9/LConn1
  Item 5 Sensor/RConn3 -- PS-Simulink Converter10/LConn1
  Item 5 Sensor/RConn4 -- PS-Simulink Converter11/LConn1
  PS-Simulink Converter13/LConn1 -- Item 4 Sensor/RConn4
  PS-Simulink Converter14/LConn1 -- Item 4 Sensor/RConn2
  PS-Simulink Converter12/LConn1 -- Item 4 Sensor/RConn3
  Item 1 Sensor/RConn2 -- PS-Simulink Converter19/LConn1
  Item 1 Sensor/RConn3 -- PS-Simulink Converter17/LConn1
  Item 1 Sensor/RConn4 -- PS-Simulink Converter18/LConn1
  Item 2 Sensor/RConn2 -- PS-Simulink Converter20/LConn1
  Item 2 Sensor/RConn3 -- PS-Simulink Converter15/LConn1
  Item 2 Sensor/RConn4 -- PS-Simulink Converter16/LConn1
  Item 3 Sensor/RConn2 -- PS-Simulink Converter23/LConn1
  Item 3 Sensor/RConn3 -- PS-Simulink Converter21/LConn1
  Item 3 Sensor/RConn4 -- PS-Simulink Converter22/LConn1
  Simscape Bus/RConn1 -- Parts/RConn1
  Simscape Bus/LConn1 -- Item 1 Sensor/RConn1
  Item 2 Sensor/RConn1 -- Simscape Bus/LConn2
  Item 3 Sensor/RConn1 -- Simscape Bus/LConn3
  Item 4 Sensor/RConn1 -- Simscape Bus/LConn4
  Simscape Bus/LConn5 -- Item 5 Sensor/RConn1
  PS-Simulink Converter1/LConn1 -- Container Inner Bottom Left Sensor/RConn2
  PS-Simulink Converter2/LConn1 -- Container Inner Bottom Left Sensor/RConn3
  PS-Simulink Converter24/LConn1 -- Container Inner Bottom Left Sensor/RConn4
  Inner Bottom Left Transform/RConn1 -- Container Inner Bottom Left Sensor/RConn1
  PS-Simulink Converter27/LConn1 -- Container Inner Top Right Sensor/RConn4
  PS-Simulink Converter26/LConn1 -- Container Inner Top Right Sensor/RConn3
  Inner Top Right Transform/RConn1 -- Container Inner Top Right Sensor/RConn1
  PS-Simulink Converter25/LConn1 -- Container Inner Top Right Sensor/RConn2

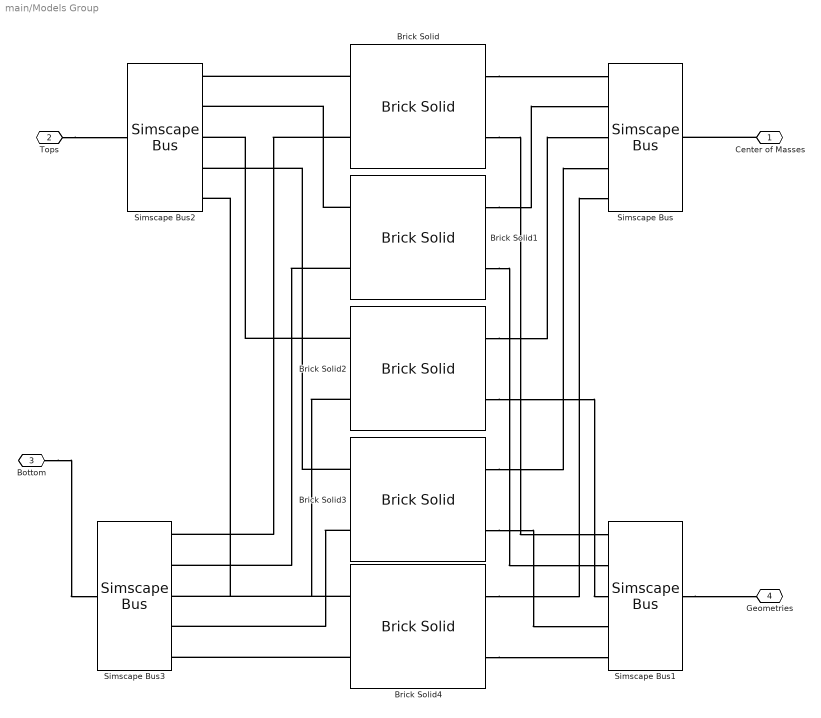
== system main/Models Group ==
  Brick Solid : sm_lib/Body Elements/Brick Solid  GraphicAmbientColor=[0.15 0.15 0.15 1.0]  BasedOnType=Density  BrickDimensions=model_dims(1, 1:3)  BrickDimensionUnits=m  CenterOfMass=[0 0 0]  CenterOfMassUnits=m  GraphicDiffuseColor=[1.0 0.0 0.0]  Density=1000  DensityUnits=kg/m^3  DoExposeReferenceFrame=on  GraphicEmissiveColor=[0.0 0.0 0.0 1.0]  ExportEntireGeometry=on  SerializedFrames=<Frames><Frame><Id>Frame1</Id><Value><Name>Top</Name><Origin><Source>GeometricFeature</Source><FeatureName>+z surface</FeatureName></Origin><PrimaryAxis><DefinedDirection>+Z</DefinedDirection><Source>ReferenceFrame</Source><SourceDirection>+Z</SourceDirection><FeatureName></FeatureName></PrimaryAxis><SecondaryAxis><DefinedDirection>+X</DefinedDirection><Source>ReferenceFrame</Source><SourceDirection>+X</SourceDirection><FeatureName></FeatureName></SecondaryAxis></Value></Frame><Frame><Id>Frame2</Id><Value><Name>Bottom</Name><Origin><Source>GeometricFeature</Source><FeatureName>-z surface</FeatureName></Origin><PrimaryAxis><DefinedDirection>+Z</DefinedDirection><Source>ReferenceFrame</Source><SourceDirection>+Z</SourceDirection><FeatureName></FeatureName></PrimaryAxis><SecondaryAxis><DefinedDirection>+X</DefinedDirection><Source>ReferenceFrame</Source><SourceDirection>+X</SourceDirection><FeatureName></FeatureName></SecondaryAxis></Value></Frame></Frames>  MarkerShape=Sphere  MarkerSize=10  GraphicType=FromGeometry  InertiaType=CalculateFromGeometry  Mass=1  MassUnits=kg  MomentsOfInertia=[1 1 1]  MomentsOfInertiaUnits=kg*m^2  GraphicOpacity=1.0  ProductsOfInertia=[0 0 0]  ProductsOfInertiaUnits=kg*m^2  GraphicShininess=75  GraphicSpecularColor=[0.5 0.5 0.5 1.0]  GraphicVisPropType=SimpleVisualProperties
  Brick Solid1 : sm_lib/Body Elements/Brick Solid  GraphicAmbientColor=[0.15 0.15 0.15 1.0]  BasedOnType=Density  BrickDimensions=model_dims(2, 1:3)  BrickDimensionUnits=m  CenterOfMass=[0 0 0]  CenterOfMassUnits=m  GraphicDiffuseColor=[0.0 0.0 1.0]  Density=1000  DensityUnits=kg/m^3  DoExposeReferenceFrame=on  GraphicEmissiveColor=[0.0 0.0 0.0 1.0]  ExportEntireGeometry=on  SerializedFrames=<Frames><Frame><Id>Frame1</Id><Value><Name>Top</Name><Origin><Source>GeometricFeature</Source><FeatureName>+z surface</FeatureName></Origin><PrimaryAxis><DefinedDirection>+Z</DefinedDirection><Source>ReferenceFrame</Source><SourceDirection>+Z</SourceDirection><FeatureName></FeatureName></PrimaryAxis><SecondaryAxis><DefinedDirection>+X</DefinedDirection><Source>ReferenceFrame</Source><SourceDirection>+X</SourceDirection><FeatureName></FeatureName></SecondaryAxis></Value></Frame><Frame><Id>Frame2</Id><Value><Name>Bottom</Name><Origin><Source>GeometricFeature</Source><FeatureName>-z surface</FeatureName></Origin><PrimaryAxis><DefinedDirection>+Z</DefinedDirection><Source>ReferenceFrame</Source><SourceDirection>+Z</SourceDirection><FeatureName></FeatureName></PrimaryAxis><SecondaryAxis><DefinedDirection>+X</DefinedDirection><Source>ReferenceFrame</Source><SourceDirection>+X</SourceDirection><FeatureName></FeatureName></SecondaryAxis></Value></Frame></Frames>  MarkerShape=Sphere  MarkerSize=10  GraphicType=FromGeometry  InertiaType=CalculateFromGeometry  Mass=1  MassUnits=kg  MomentsOfInertia=[1 1 1]  MomentsOfInertiaUnits=kg*m^2  GraphicOpacity=1.0  ProductsOfInertia=[0 0 0]  ProductsOfInertiaUnits=kg*m^2  GraphicShininess=75  GraphicSpecularColor=[0.5 0.5 0.5 1.0]  GraphicVisPropType=SimpleVisualProperties
  Brick Solid2 : sm_lib/Body Elements/Brick Solid  GraphicAmbientColor=[0.15 0.15 0.15 1.0]  BasedOnType=Density  BrickDimensions=model_dims(3, 1:3)  BrickDimensionUnits=m  CenterOfMass=[0 0 0]  CenterOfMassUnits=m  GraphicDiffuseColor=[0.0 1.0 0.0]  Density=1000  DensityUnits=kg/m^3  DoExposeReferenceFrame=on  GraphicEmissiveColor=[0.0 0.0 0.0 1.0]  ExportEntireGeometry=on  SerializedFrames=<Frames><Frame><Id>Frame1</Id><Value><Name>Top</Name><Origin><Source>GeometricFeature</Source><FeatureName>+z surface</FeatureName></Origin><PrimaryAxis><DefinedDirection>+Z</DefinedDirection><Source>ReferenceFrame</Source><SourceDirection>+Z</SourceDirection><FeatureName></FeatureName></PrimaryAxis><SecondaryAxis><DefinedDirection>+X</DefinedDirection><Source>ReferenceFrame</Source><SourceDirection>+X</SourceDirection><FeatureName></FeatureName></SecondaryAxis></Value></Frame><Frame><Id>Frame2</Id><Value><Name>Bottom</Name><Origin><Source>GeometricFeature</Source><FeatureName>-z surface</FeatureName></Origin><PrimaryAxis><DefinedDirection>+Z</DefinedDirection><Source>ReferenceFrame</Source><SourceDirection>+Z</SourceDirection><FeatureName></FeatureName></PrimaryAxis><SecondaryAxis><DefinedDirection>+X</DefinedDirection><Source>ReferenceFrame</Source><SourceDirection>+X</SourceDirection><FeatureName></FeatureName></SecondaryAxis></Value></Frame></Frames>  MarkerShape=Sphere  MarkerSize=10  GraphicType=FromGeometry  InertiaType=CalculateFromGeometry  Mass=1  MassUnits=kg  MomentsOfInertia=[1 1 1]  MomentsOfInertiaUnits=kg*m^2  GraphicOpacity=1.0  ProductsOfInertia=[0 0 0]  ProductsOfInertiaUnits=kg*m^2  GraphicShininess=75  GraphicSpecularColor=[0.5 0.5 0.5 1.0]  GraphicVisPropType=SimpleVisualProperties
  Brick Solid3 : sm_lib/Body Elements/Brick Solid  GraphicAmbientColor=[0.15 0.15 0.15 1.0]  BasedOnType=Density  BrickDimensions=model_dims(4, 1:3)  BrickDimensionUnits=m  CenterOfMass=[0 0 0]  CenterOfMassUnits=m  GraphicDiffuseColor=[1.0 0.0 0.8]  Density=1000  DensityUnits=kg/m^3  DoExposeReferenceFrame=on  GraphicEmissiveColor=[0.0 0.0 0.0 1.0]  ExportEntireGeometry=on  SerializedFrames=<Frames><Frame><Id>Frame1</Id><Value><Name>Top</Name><Origin><Source>GeometricFeature</Source><FeatureName>+z surface</FeatureName></Origin><PrimaryAxis><DefinedDirection>+Z</DefinedDirection><Source>ReferenceFrame</Source><SourceDirection>+Z</SourceDirection><FeatureName></FeatureName></PrimaryAxis><SecondaryAxis><DefinedDirection>+X</DefinedDirection><Source>ReferenceFrame</Source><SourceDirection>+X</SourceDirection><FeatureName></FeatureName></SecondaryAxis></Value></Frame><Frame><Id>Frame2</Id><Value><Name>Bottom</Name><Origin><Source>GeometricFeature</Source><FeatureName>-z surface</FeatureName></Origin><PrimaryAxis><DefinedDirection>+Z</DefinedDirection><Source>ReferenceFrame</Source><SourceDirection>+Z</SourceDirection><FeatureName></FeatureName></PrimaryAxis><SecondaryAxis><DefinedDirection>+X</DefinedDirection><Source>ReferenceFrame</Source><SourceDirection>+X</SourceDirection><FeatureName></FeatureName></SecondaryAxis></Value></Frame></Frames>  MarkerShape=Sphere  MarkerSize=10  GraphicType=FromGeometry  InertiaType=CalculateFromGeometry  Mass=1  MassUnits=kg  MomentsOfInertia=[1 1 1]  MomentsOfInertiaUnits=kg*m^2  GraphicOpacity=1.0  ProductsOfInertia=[0 0 0]  ProductsOfInertiaUnits=kg*m^2  GraphicShininess=75  GraphicSpecularColor=[0.5 0.5 0.5 1.0]  GraphicVisPropType=SimpleVisualProperties
  Brick Solid4 : sm_lib/Body Elements/Brick Solid  GraphicAmbientColor=[0.15 0.15 0.15 1.0]  BasedOnType=Density  BrickDimensions=model_dims(5, 1:3)  BrickDimensionUnits=m  CenterOfMass=[0 0 0]  CenterOfMassUnits=m  GraphicDiffuseColor=[1.0 0.6 0.0]  Density=1000  DensityUnits=kg/m^3  DoExposeReferenceFrame=on  GraphicEmissiveColor=[0.0 0.0 0.0 1.0]  ExportEntireGeometry=on  SerializedFrames=<Frames><Frame><Id>Frame1</Id><Value><Name>Top</Name><Origin><Source>GeometricFeature</Source><FeatureName>+z surface</FeatureName></Origin><PrimaryAxis><DefinedDirection>+Z</DefinedDirection><Source>ReferenceFrame</Source><SourceDirection>+Z</SourceDirection><FeatureName></FeatureName></PrimaryAxis><SecondaryAxis><DefinedDirection>+X</DefinedDirection><Source>ReferenceFrame</Source><SourceDirection>+X</SourceDirection><FeatureName></FeatureName></SecondaryAxis></Value></Frame><Frame><Id>Frame2</Id><Value><Name>Bottom</Name><Origin><Source>GeometricFeature</Source><FeatureName>-z surface</FeatureName></Origin><PrimaryAxis><DefinedDirection>+Z</DefinedDirection><Source>ReferenceFrame</Source><SourceDirection>+Z</SourceDirection><FeatureName></FeatureName></PrimaryAxis><SecondaryAxis><DefinedDirection>+X</DefinedDirection><Source>ReferenceFrame</Source><SourceDirection>+X</SourceDirection><FeatureName></FeatureName></SecondaryAxis></Value></Frame></Frames>  MarkerShape=Sphere  MarkerSize=10  GraphicType=FromGeometry  InertiaType=CalculateFromGeometry  Mass=1  MassUnits=kg  MomentsOfInertia=[1 1 1]  MomentsOfInertiaUnits=kg*m^2  GraphicOpacity=1.0  ProductsOfInertia=[0 0 0]  ProductsOfInertiaUnits=kg*m^2  GraphicShininess=75  GraphicSpecularColor=[0.5 0.5 0.5 1.0]  GraphicVisPropType=SimpleVisualProperties
  Simscape Bus{,1..3} (4 alike) : SimscapeBus  HierarchyStrings=Part1;Part2;Part3;Part4;Part5
  Center of Masses : PMIOPort  Side=Right
  Tops : PMIOPort  Port=2  Side=Left
  Bottom : PMIOPort  Port=3  Side=Left
  Geometries : PMIOPort  Port=4  Side=Right
  connections:
  Brick Solid/RConn1 -- Simscape Bus/LConn1
  Brick Solid1/RConn1 -- Simscape Bus/LConn2
  Brick Solid2/RConn1 -- Simscape Bus/LConn3
  Brick Solid3/RConn1 -- Simscape Bus/LConn4
  Brick Solid4/RConn1 -- Simscape Bus/LConn5
  Brick Solid/RConn2 -- Simscape Bus1/LConn1
  Brick Solid1/RConn2 -- Simscape Bus1/LConn2
  Brick Solid2/RConn2 -- Simscape Bus1/LConn3
  Brick Solid3/RConn2 -- Simscape Bus1/LConn4
  Brick Solid4/RConn2 -- Simscape Bus1/LConn5
  Center of Masses/RConn1 -- Simscape Bus/RConn1
  Simscape Bus1/RConn1 -- Geometries/RConn1
  Bottom/RConn1 -- Simscape Bus3/RConn1
  Tops/RConn1 -- Simscape Bus2/RConn1
  Brick Solid/LConn1 -- Simscape Bus2/LConn1
  Brick Solid1/LConn1 -- Simscape Bus2/LConn2
  Brick Solid2/LConn1 -- Simscape Bus2/LConn3
  Brick Solid/LConn2 -- Simscape Bus3/LConn1
  Brick Solid1/LConn2 -- Simscape Bus3/LConn2
  Brick Solid2/LConn2 -- Simscape Bus3/LConn3
  Brick Solid3/LConn2 -- Simscape Bus3/LConn4
  Brick Solid4/LConn2 -- Simscape Bus3/LConn5
  Brick Solid3/LConn1 -- Simscape Bus2/LConn4
  Brick Solid4/LConn1 -- Simscape Bus2/LConn5
